simulink model "correlated_binomial_noise"  (R2022b)
settings: Solver=FixedStepAuto  StartTime=0.0  StopTime=10.0  FixedStep=.1  RelTol=1e-3
libraries: commrandsrc3 x1
settings Model: Creator=Sajjad  LastModifiedBy=Sajjad

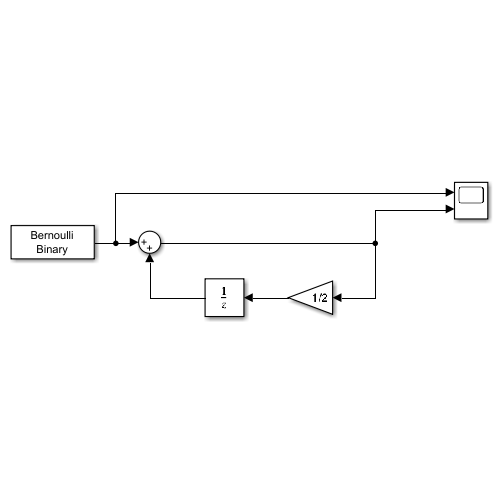
[thumbnail: Simulink's stored preview of the top-level diagram]
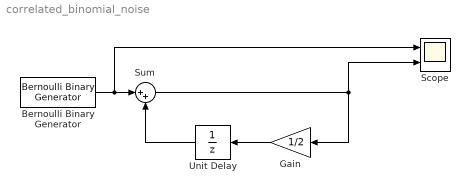
== system correlated_binomial_noise ==
  Bernoulli Binary Generator : commrandsrc3/Bernoulli Binary Generator  ProbabilityOfZero=0.5  SeedSource=Auto  Seed=0  SampleTime=-1  SamplesPerFrame=1  OutputDataType=double  SimulateUsing=Code generation
  Gain : Gain  Gain=1/2
  Scope : Scope  NumInputPorts=2
  Sum : Sum  Inputs=|++
  Unit Delay : UnitDelay  SampleTime=-1  HasFrameUpgradeWarning=on
  wires:
  Gain/1 -> Unit Delay/1
  Unit Delay/1 -> Sum/2
  Bernoulli Binary Generator/1 -> Scope/1, Sum/1
  Sum/1 -> Gain/1, Scope/2
